simulink model "DM_Encoder_Decoder"  (R2024b)
settings: Solver=VariableStepAuto  StartTime=0.0  StopTime=10.0  RelTol=1e-3
libraries: dspfdesign x1, dspsigops x1
settings Model: Creator=white  LastModifiedBy=white

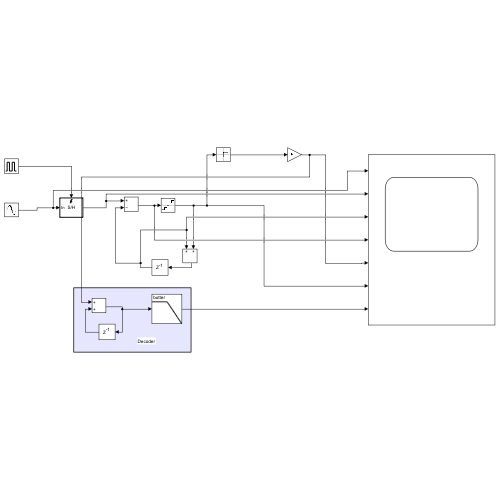
[thumbnail: Simulink's stored preview of the top-level diagram]
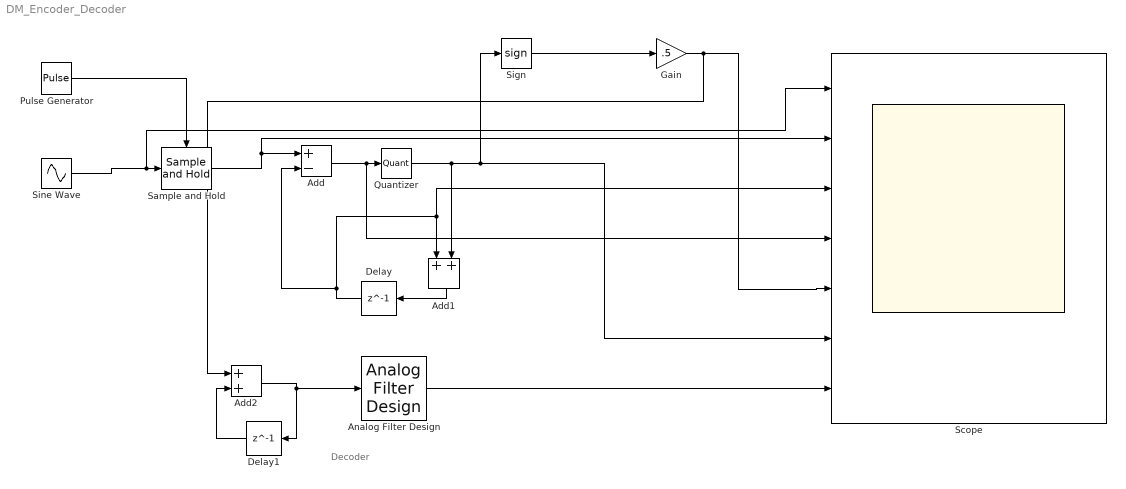
== system DM_Encoder_Decoder ==
  note: Decoder
  Add : Sum  Inputs=+-
  Add1 : Sum
  Add2 : Sum
  Analog Filter Design : dspfdesign/Analog Filter Design  method=Butterworth  filttype=Lowpass  N=8  Wlo=2*pi*2  Whi=80  Rp=2  Rs=40
  Delay : Delay  DelayLength=1  InitialCondition=0
  Delay1 : Delay  DelayLength=1  InitialCondition=0
  Gain : Gain  Gain=.5
  Pulse Generator : DiscretePulseGenerator  PulseType=Time based  Amplitude=5  Period=1/40  PulseWidth=5
  Quantizer : Quantizer
  Sample and Hold : dspsigops/Sample and Hold  trig=Rising edge  initCond=0  latchinput=off
  Scope : Scope  NumInputPorts=7
  Sign : Signum
  Sine Wave : Sin  Amplitude=5  Frequency=2*pi*2  SampleTime=1/10000
  wires:
  Pulse Generator/1 -> Sample and Hold/Trigger
  Sine Wave/1 -> Scope/1, Sample and Hold/1
  Sample and Hold/1 -> Scope/2, Add/1
  Add/1 -> Scope/4, Quantizer/1
  Add1/1 -> Delay/1
  Quantizer/1 -> Add1/2, Scope/6, Sign/1
  Delay/1 -> Add/2, Scope/3, Add1/1
  Gain/1 -> Add2/1, Scope/5
  Sign/1 -> Gain/1
  Delay1/1 -> Add2/2
  Add2/1 -> Delay1/1, Analog Filter Design/1
  Analog Filter Design/1 -> Scope/7
